simulink model "Part2"  (R2020a)
settings: Solver=VariableStepAuto  StartTime=0.0  StopTime=75  RelTol=1e-3
values from neighbouring files (symbols this model uses):
  b = 50    [Script1.m]
  m = 1000    [Script1.m]
  V = 90    [Script1.m]
libraries: cstblocks x1
settings Model: Creator=maxen  LastModifiedBy=maxen

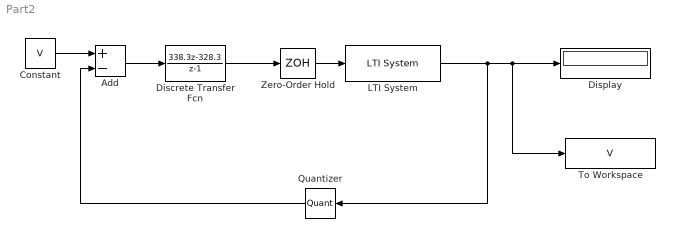
== system Part2 ==
  Add : Sum  Inputs=+-
  Constant : Constant  Value=V
  Discrete Transfer Fcn : DiscreteTransferFcn  Numerator=[338.3 -328.3]  Denominator=[1 -1]  SampleTime=0.6
  Display : Display
  LTI System : cstblocks/LTI System  sys=tf(1,[m b])  IC=[]
  Quantizer : Quantizer  QuantizationInterval=0.25
  To Workspace : ToWorkspace  VariableName=V  SampleTime=-1
  Zero-Order Hold : ZeroOrderHold  SampleTime=-1
  wires:
  Constant/1 -> Add/1
  LTI System/1 -> Quantizer/1, To Workspace/1, Display/1
  Add/1 -> Discrete Transfer Fcn/1
  Discrete Transfer Fcn/1 -> Zero-Order Hold/1
  Zero-Order Hold/1 -> LTI System/1
  Quantizer/1 -> Add/2
